simulink model "StateflowConcepts"  (R2019a)
settings: Solver=FixedStepAuto  StartTime=0.0  StopTime=10.0  FixedStep=0.01  RelTol=1e-3
settings Model: Creator=vk09330  LastModifiedBy=vk09330
settings DataIOCC: ReturnWorkspaceOutputs=off
settings DebuggingCC: ArithmeticOperatorsInVariantConditions=warning
settings SFSimCC: SimUseLocalCustomCode=off
settings RTWCC: RTWUseLocalCustomCode=off
settings ConfigComp: CovEnable=on  RecordCoverage=on  CovModelRefEnable=on

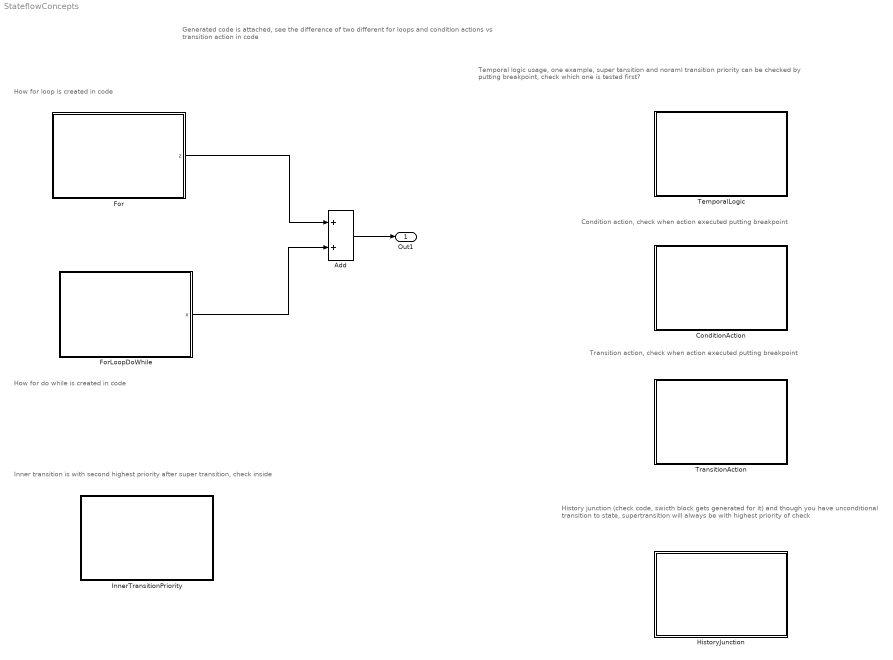
== system StateflowConcepts ==
  note: Generated code is attached, see the difference of two different for loops and condition actions vs transition action in code
  note: Temporal logic usage, one example, super tansition and noraml transition priority can be checked
      | by putting breakpoint, check which one is tested first?
  note: Condition action, check when action executed putting breakpoint
  note: Transition action, check when action executed putting breakpoint
  note: How for loop is created in code
  note: How for do while is created in code
  note: Inner transition is with second highest priority after super transition, check inside
  note: History junction (check code, swicth block gets generated for it)
      | and though you have unconditional transition to state, supertransition
      | will always be with highest priority of check
  Add : Sum
  ConditionAction : Stateflow chart  TreatAsAtomicUnit=on
  For : Stateflow chart  TreatAsAtomicUnit=on
  ForLoopDoWhile : Stateflow chart  TreatAsAtomicUnit=on
  HistoryJunction : Stateflow chart  TreatAsAtomicUnit=on
  InnerTransitionPriority : Stateflow chart  TreatAsAtomicUnit=on
  TemporalLogic : Stateflow chart  TreatAsAtomicUnit=on
  TransitionAction : Stateflow chart  TreatAsAtomicUnit=on
  Out1 : Outport
  wires:
  For/1(z) -> Add/1
  ForLoopDoWhile/1(x) -> Add/2
  Add/1 -> Out1/1

== stateflow chart StateflowConcepts/TemporalLogic ==
  state MainState
    state State1
      en: a = 0;
      du: a = 5;
    state State2
      entry: a = 10;
      du: a = a + 1;
    (default) -> State1
    State1 -> State2 : [after(50, msec)]
  (default) -> (junction 27) : {a=0;}
  MainState -> (junction 27) : [a>10]
  (junction 27) -> (junction 29)
  (junction 29) -> (junction 31) : {a=a+1;}
  (junction 31) -> (junction 29) [order 1] : [a<5]
  (junction 31) -> MainState [order 2]
  data: a local

== stateflow chart StateflowConcepts/For ==
  state XYZW
  (default) -> XYZW
  XYZW -> (junction 31) : % WhileLoop
  (junction 25) -> (junction 33) [order 1] : [a<10]
  (junction 33) -> (junction 28) : {z=10;} %check
  (junction 31) -> (junction 25) : {a=0;}
  (junction 28) -> (junction 25) : {a=a+1;}
  (junction 25) -> (junction 30) [order 2]
  data: a local; z output

== stateflow chart StateflowConcepts/ForLoopDoWhile ==
  state ABCD
    entry: x=10;
  (default) -> ABCD
  (junction 1) -> (junction 4) : {x=x+1;}
  ABCD -> (junction 1)
  (junction 4) -> (junction 1) [order 1] : [x<5]
  (junction 4) -> (junction 8) [order 2]
  data: x output

== stateflow chart StateflowConcepts/ConditionAction ==
  state MainState
    state State1
      en: a = 0;
      du: a = a+1;
    state State2
      entry: a = 10;
      du: a = a + 1;
    (default) -> State1
    State1 -> State2 : [a>2]{a=5;}
    State2 -> State1 : [a>12]{a=5;}
  data: a local

== stateflow chart StateflowConcepts/TransitionAction ==
  state MainState
    state State1
      en: a = 0;
      du: a = a+1;
    state State2
      entry: a = 10;
      du: a = a + 1;
    (default) -> State1
    State1 -> State2 : [a>2]/{a=5;}
    State2 -> State1 : [a>12]/{a=5;}
  data: a local

== stateflow chart StateflowConcepts/InnerTransitionPriority ==
  state MainState
    state State1
      en: a = 0;
      du: a = a+1;
      ex: a = 100;
    state State2
      entry: a = 10;
      du: a = a + 1;
    (default) -> State1
    State1 -> State2 : [a>1]
  MainState -> (junction 27) : [a>10]
  (junction 27) -> (junction 29) : {a=0;}
  (junction 29) -> (junction 31) : {a=a+1;}
  (junction 31) -> (junction 29) [order 1] : [a<5]
  (junction 31) -> MainState [order 2]
  data: a local

== stateflow chart StateflowConcepts/HistoryJunction ==
  state MainState
    (history)
    state State2
      entry: a = 10;
      du: a = a + 1;
    state State1
      en: a = 0;
      du: a = a+1;
    state State3
    (default) -> State1 : { b=0;}
    State1 -> State2 : [a>1]
    (junction 63) -> State1
    State2 -> State3 : [a>10 && b==0]
    State3 -> (junction 63) : {b=1;}
  MainState -> (junction 27) : [a>10 && b==1]
  (junction 27) -> (junction 29) : {a=0;}
  (junction 29) -> (junction 31) : {a=a+1;}
  (junction 31) -> (junction 29) [order 1] : [a<5]
  (junction 31) -> MainState [order 2]
  data: a local; b local
